simulink model "Test_1_2018a"  (Simulink 9.1)
settings: Solver=VariableStepAuto  StartTime=0.0  StopTime=32  RelTol=1e-3
values from neighbouring files (symbols this model uses):
  CdA = 0.08    [lqrparameters.m]
  d = 0.086    [lqrparameters.m]
  g = 9.81    [lqrparameters.m]
  Ix = 0.00025    [lqrparameters.m]
  Iy = 0.000432    [lqrparameters.m]
  Iz = 0.0003738    [lqrparameters.m]
  kfay = 0.01    [lqrparameters.m]
  kfaz = 0.01    [lqrparameters.m]
  kftx = 0.1    [lqrparameters.m]
  kfty = 0.1    [lqrparameters.m]
  kftz = 0.1    [lqrparameters.m]
  m = 0.18    [lqrparameters.m]
  rho = 1.225    [lqrparameters.m]
undefined symbols (not defined in the file or in its folder): DiscIntNeverNeededParam
libraries: peSlidingModeController x6, aerolibutil x1, sharedtransform x1, aerolibwind2 x1
settings Model: Creator=Ayush  LastModifiedBy=Rishabh Verma
settings DataIOCC: SaveFormat=Dataset
settings OptimizationCC: LifeSpan=auto
settings DebuggingCC: UnderspecifiedInitializationDetection=Simplified  MergeDetectMultiDrivingBlocksExec=error  LibraryContextMissingDiagnostic=warning  SFUnexpectedBacktrackingDiag=error  SFNoUnconditionalDefaultTransitionDiag=error  SFExecutionAtInitializationDiag=warning
settings HardwareCC: ProdBitPerPointer=64  ProdBitPerSizeT=64  ProdBitPerPtrDiffT=64  ProdLargestAtomicFloat=Float  ProdIntDivRoundTo=Zero  ProdEndianess=LittleEndian  ProdWordSize=64  ProdHWDeviceType=Intel->x86-64 (Windows64)
settings ModelReferenceCC: PropagateSignalLabelsOutOfModel=on
settings SFSimCC: SimUseLocalCustomCode=on
settings RTWCC: RTWUseLocalCustomCode=on
settings CodeAppCC: StateflowObjectComments=off
settings GRTTargetCC: TargetLangStandard=C99 (ISO)  CombineOutputUpdateFcns=on  GRTInterface=off
settings ConfigComp: CovMetricSettings=dwe  CovHtmlReporting=off  CovSaveCumulativeToWorkspaceVar=off  CovSaveSingleToWorkspaceVar=off  CovExternalEMLEnable=on

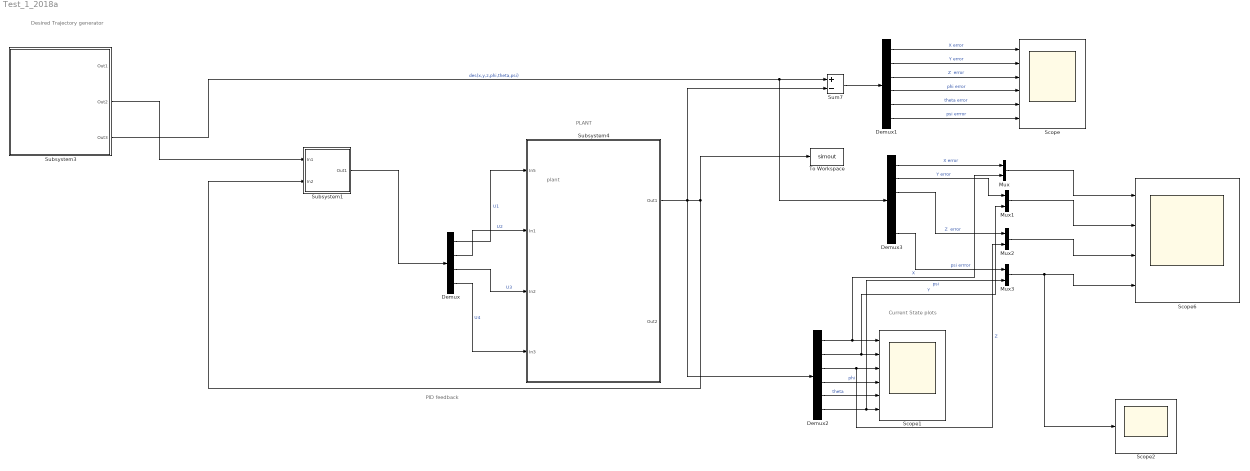
== system Test_1_2018a ==
  note: Desired Trajectory
      | generator
  note: PID feedback
  note: PLANT
  note: Current State
      | plots
  note: plant
  Demux : Demux
  Demux1 : Demux  Outputs=6
  Demux2 : Demux  Outputs=6
  Demux3 : Demux  Outputs=6
  Mux{,1..3} (4 alike) : Mux  Inputs=2
  Scope : Scope  NumInputPorts=6
  Scope1 : Scope  NumInputPorts=6
  Scope2 : Scope
  Scope6 : Scope  NumInputPorts=4
  Subsystem1 : Subsystem
  Subsystem3 : Subsystem
  Subsystem4 : Subsystem
  Sum7 : Sum  Inputs=+-
  To Workspace : ToWorkspace  VariableName=simout  SampleTime=0.01
  wires:
  Subsystem3/3(Out3) -> Demux3/1, Sum7/1  "des(x,y,z,phi,theta,psi)"
  Demux1/6 -> Scope/6  "psi errror"
  Demux1/5 -> Scope/5  "theta error"
  Demux1/2 -> Scope/2  "Y error"
  Sum7/1 -> Demux1/1
  Subsystem4/1(Out1) -> Sum7/2, Demux2/1, Subsystem1/2(In2), To Workspace/1
  Demux1/1 -> Scope/1  "X error"
  Demux2/4 -> Scope1/4  "phi"
  Demux2/1 -> Mux/2, Scope1/1  "X"
  Demux2/5 -> Scope1/5  "theta"
  Demux2/6 -> Mux3/2, Scope1/6  "psi"
  Demux2/3 -> Mux2/2, Scope1/3  "Z"
  Demux1/3 -> Scope/3  "Z  error"
  Demux2/2 -> Mux1/2, Scope1/2  "Y"
  Demux1/4 -> Scope/4  "phi error"
  Demux3/1 -> Mux/1  "X error"
  Demux3/2 -> Mux1/1  "Y error"
  Demux3/3 -> Mux2/1  "Z  error"
  Demux3/6 -> Mux3/1  "psi errror"
  Mux/1 -> Scope6/1
  Mux1/1 -> Scope6/2
  Mux2/1 -> Scope6/3
  Mux3/1 -> Scope2/1, Scope6/4
  Demux/1 -> Subsystem4/1(In5)  "U1"
  Demux/2 -> Subsystem4/2(In1)  "U2"
  Demux/3 -> Subsystem4/3(In2)  "U3"
  Demux/4 -> Subsystem4/4(In3)  "U4"
  Subsystem3/2(Out2) -> Subsystem1/1(In1)
  Subsystem1/1(Out1) -> Demux/1

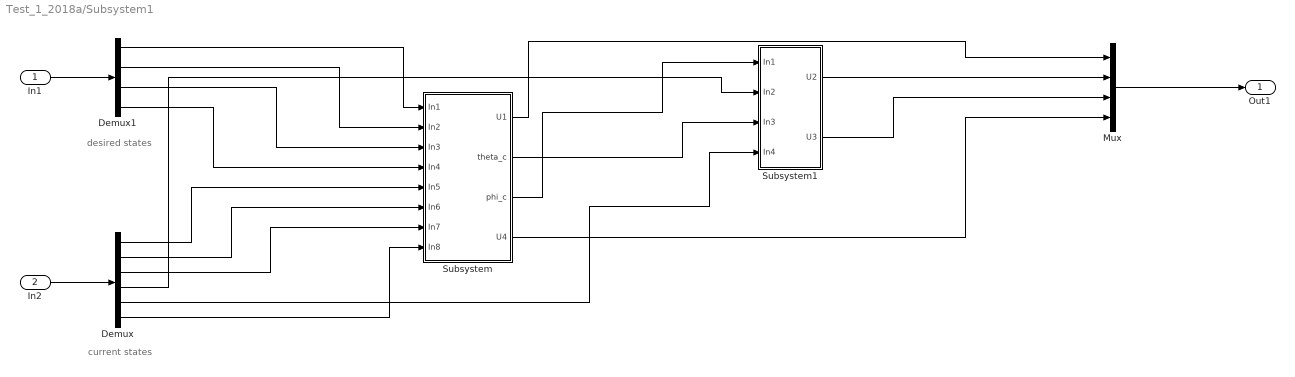
== system Test_1_2018a/Subsystem1 ==
  note: current states
  note: desired states
  In1 : Inport
  In2 : Inport  Port=2
  Demux : Demux  Outputs=6
  Demux1 : Demux
  Mux : Mux
  Subsystem : Subsystem
  Subsystem1 : Subsystem
  Out1 : Outport
  wires:
  Mux/1 -> Out1/1
  In2/1 -> Demux/1
  In1/1 -> Demux1/1
  Demux1/1 -> Subsystem/1(In1)
  Demux1/2 -> Subsystem/2(In2)
  Demux1/3 -> Subsystem/3(In3)
  Demux1/4 -> Subsystem/4(In4)
  Demux/1 -> Subsystem/5(In5)
  Demux/2 -> Subsystem/6(In6)
  Demux/3 -> Subsystem/7(In7)
  Demux/6 -> Subsystem/8(In8)
  Subsystem/2(theta_c) -> Subsystem1/3(In3)
  Demux/4 -> Subsystem1/2(In2)
  Demux/5 -> Subsystem1/4(In4)
  Subsystem/3(phi_c) -> Subsystem1/1(In1)
  Subsystem1/1(U2) -> Mux/2
  Subsystem/1(U1) -> Mux/1
  Subsystem/4(U4) -> Mux/4
  Subsystem1/2(U3) -> Mux/3

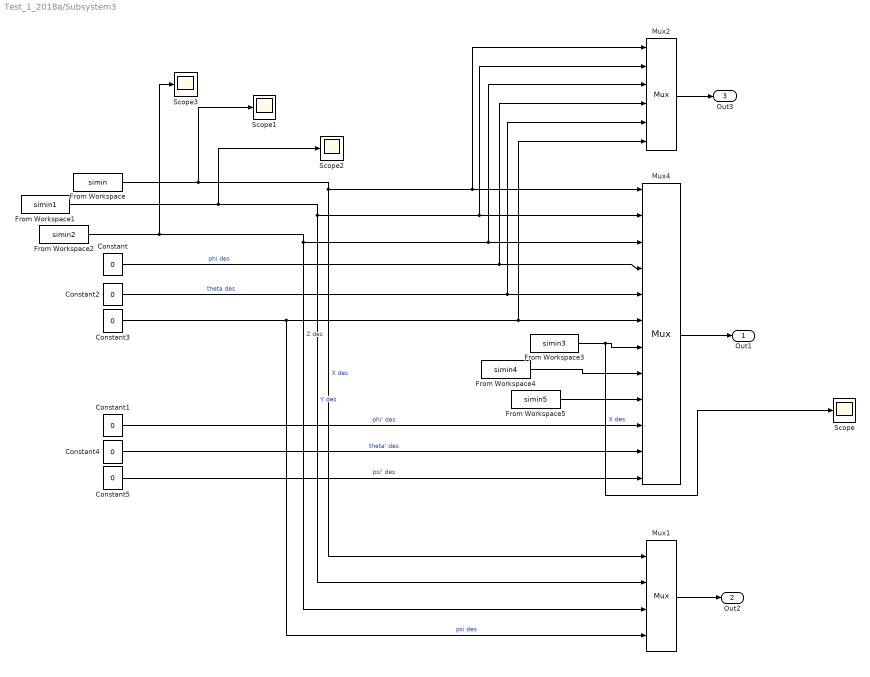
== system Test_1_2018a/Subsystem3 ==
  Constant{,1..5} (6 alike) : Constant  Value=0
  From Workspace : FromWorkspace  VariableName=simin  SampleTime=0
  From Workspace1 : FromWorkspace  VariableName=simin1  SampleTime=0
  From Workspace2 : FromWorkspace  VariableName=simin2  SampleTime=0
  From Workspace3 : FromWorkspace  VariableName=simin3  SampleTime=0
  From Workspace4 : FromWorkspace  VariableName=simin4  SampleTime=0
  From Workspace5 : FromWorkspace  VariableName=simin5  SampleTime=0
  Mux1 : Mux
      settings: DisplayOption=signals
  Mux2 : Mux  Inputs=6
      settings: DisplayOption=signals
  Mux4 : Mux  Inputs=12
      settings: DisplayOption=signals
  Scope{,1..3} (4 alike) : Scope
  Out1 : Outport
  Out2 : Outport  Port=2
  Out3 : Outport  Port=3
  wires:
  From Workspace/1 -> Scope1/1, Mux1/1, Mux2/1, Mux4/1  "X des"
  Constant1/1 -> Mux4/10  "phi' des"
  From Workspace1/1 -> Scope2/1, Mux1/2, Mux2/2, Mux4/2  "Y des"
  Constant2/1 -> Mux2/5, Mux4/5  "theta des"
  Constant/1 -> Mux2/4, Mux4/4  "phi des"
  Constant5/1 -> Mux4/12  "psi' des"
  From Workspace2/1 -> Scope3/1, Mux1/3, Mux2/3, Mux4/3  "Z des"
  Constant3/1 -> Mux1/4, Mux2/6, Mux4/6  "psi des"
  Constant4/1 -> Mux4/11  "theta' des"
  Mux1/1 -> Out2/1
  Mux4/1 -> Out1/1
  Mux2/1 -> Out3/1
  From Workspace4/1 -> Mux4/8
  From Workspace5/1 -> Mux4/9
  From Workspace3/1 -> Scope/1, Mux4/7  "X des"

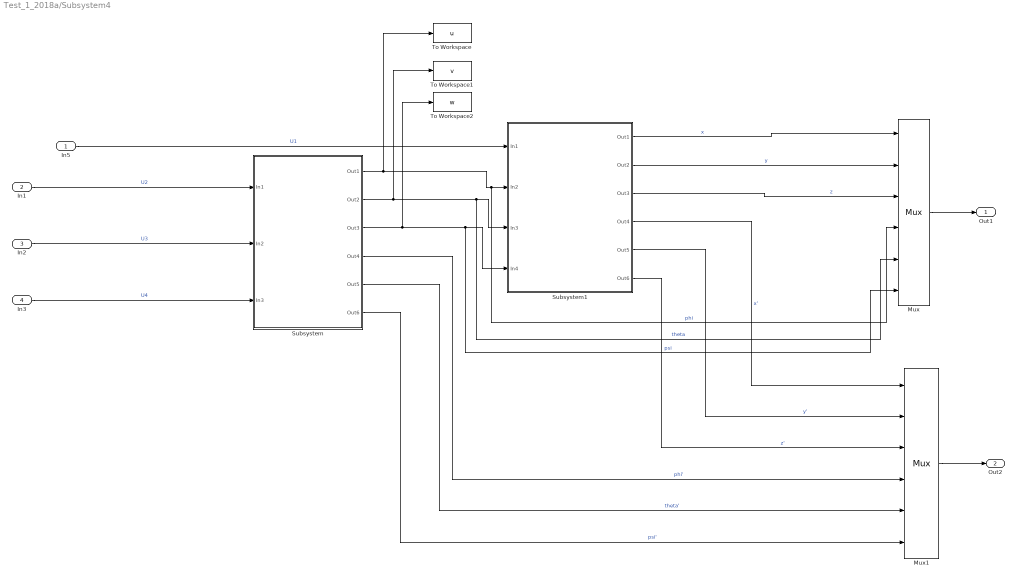
== system Test_1_2018a/Subsystem4 ==
  In5 : Inport
  In1 : Inport  Port=2
  In2 : Inport  Port=3
  In3 : Inport  Port=4
  Mux : Mux  Inputs=6
      settings: DisplayOption=signals
  Mux1 : Mux  Inputs=6
      settings: DisplayOption=signals
  Subsystem : Subsystem
  Subsystem1 : Subsystem
  To Workspace : ToWorkspace  VariableName=u  SaveFormat=Timeseries  SampleTime=-1
  To Workspace1 : ToWorkspace  VariableName=v  SaveFormat=Timeseries  SampleTime=-1
  To Workspace2 : ToWorkspace  VariableName=w  SaveFormat=Timeseries  SampleTime=-1
  Out1 : Outport
  Out2 : Outport  Port=2
  wires:
  Subsystem1/2(Out2) -> Mux/2  "y"
  Subsystem/1(Out1) -> To Workspace/1, Subsystem1/2(In2), Mux/4  "phi"
  Subsystem1/1(Out1) -> Mux/1  "x"
  In1/1 -> Subsystem/1(In1)  "U2"
  Subsystem/3(Out3) -> To Workspace2/1, Mux/6, Subsystem1/4(In4)  "psi"
  In3/1 -> Subsystem/3(In3)  "U4"
  Subsystem1/3(Out3) -> Mux/3  "z"
  Subsystem1/6(Out6) -> Mux1/3  "z'"
  In2/1 -> Subsystem/2(In2)  "U3"
  In5/1 -> Subsystem1/1(In1)  "U1"
  Subsystem1/4(Out4) -> Mux1/1  "x'"
  Subsystem1/5(Out5) -> Mux1/2  "y'"
  Subsystem/2(Out2) -> To Workspace1/1, Mux/5, Subsystem1/3(In3)  "theta"
  Subsystem/4(Out4) -> Mux1/4  "phi'"
  Subsystem/5(Out5) -> Mux1/5  "theta'"
  Subsystem/6(Out6) -> Mux1/6  "psi'"
  Mux/1 -> Out1/1
  Mux1/1 -> Out2/1

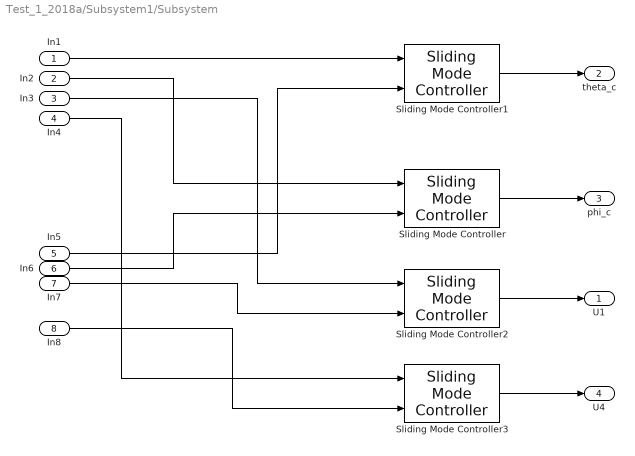
== system Test_1_2018a/Subsystem1/Subsystem ==
  In1 : Inport
  In2 : Inport  Port=2
  In3 : Inport  Port=3
  In4 : Inport  Port=4
  In5 : Inport  Port=5
  In6 : Inport  Port=6
  In7 : Inport  Port=7
  In8 : Inport  Port=8
  Sliding Mode Controller{,1..3} (4 alike) : peSlidingModeController/Sliding Mode Controller  h=0.2  up=10  lo=-10  Ts=-1
  U1 : Outport
  theta_c : Outport  Port=2
  phi_c : Outport  Port=3
  U4 : Outport  Port=4
  wires:
  In6/1 -> Sliding Mode Controller/2
  In1/1 -> Sliding Mode Controller1/1
  In7/1 -> Sliding Mode Controller2/2
  In5/1 -> Sliding Mode Controller1/2
  In4/1 -> Sliding Mode Controller3/1
  In2/1 -> Sliding Mode Controller/1
  In3/1 -> Sliding Mode Controller2/1
  In8/1 -> Sliding Mode Controller3/2
  Sliding Mode Controller2/1 -> U1/1
  Sliding Mode Controller3/1 -> U4/1
  Sliding Mode Controller1/1 -> theta_c/1
  Sliding Mode Controller/1 -> phi_c/1

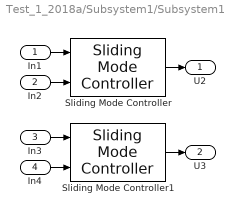
== system Test_1_2018a/Subsystem1/Subsystem1 ==
  In1 : Inport
  In2 : Inport  Port=2
  In3 : Inport  Port=3
  In4 : Inport  Port=4
  Sliding Mode Controller : peSlidingModeController/Sliding Mode Controller  h=0.2  up=10  lo=-10  Ts=-1
  Sliding Mode Controller1 : peSlidingModeController/Sliding Mode Controller  h=0.2  up=10  lo=-10  Ts=-1
  U2 : Outport
  U3 : Outport  Port=2
  wires:
  Sliding Mode Controller1/1 -> U3/1
  In2/1 -> Sliding Mode Controller/2
  In3/1 -> Sliding Mode Controller1/1
  In4/1 -> Sliding Mode Controller1/2
  Sliding Mode Controller/1 -> U2/1
  In1/1 -> Sliding Mode Controller/1

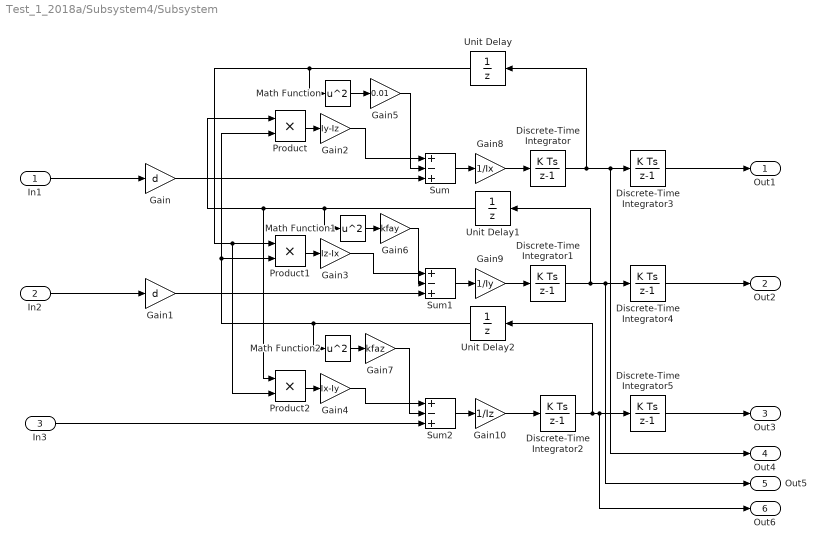
== system Test_1_2018a/Subsystem4/Subsystem ==
  In1 : Inport
  In2 : Inport  Port=2
  In3 : Inport  Port=3
  Discrete-Time Integrator{,1..5} (6 alike) : DiscreteIntegrator  SampleTime=-1  ICPrevOutput=DiscIntNeverNeededParam  ICPrevScaledInput=DiscIntNeverNeededParam
  Gain : Gain  Gain=d
  Gain1 : Gain  Gain=d
  Gain10 : Gain  Gain=1/Iz
  Gain2 : Gain  Gain=Iy-Iz
  Gain3 : Gain  Gain=Iz-Ix
  Gain4 : Gain  Gain=Ix-Iy
  Gain5 : Gain  Gain=0.01
  Gain6 : Gain  Gain=kfay
  Gain7 : Gain  Gain=kfaz
  Gain8 : Gain  Gain=1/Ix
  Gain9 : Gain  Gain=1/Iy
  Math Function : Math  Operator=square  SaturateOnIntegerOverflow=on
  Math Function1 : Math  Operator=square  SaturateOnIntegerOverflow=on
  Math Function2 : Math  Operator=square  SaturateOnIntegerOverflow=on
  Product : Product
  Product1 : Product
  Product2 : Product
  Sum : Sum  Inputs=+-+
  Sum1 : Sum  Inputs=+-+
  Sum2 : Sum  Inputs=+-+
  Unit Delay : UnitDelay  SampleTime=0.001
  Unit Delay1 : UnitDelay  SampleTime=0.001
  Unit Delay2 : UnitDelay  SampleTime=0.001
  Out1 : Outport
  Out2 : Outport  Port=2
  Out3 : Outport  Port=3
  Out4 : Outport  Port=4
  Out5 : Outport  Port=5
  Out6 : Outport  Port=6
  wires:
  Unit Delay/1 -> Math Function/1, Product2/2, Product1/1
  Discrete-Time Integrator1/1 -> Out5/1, Discrete-Time Integrator4/1, Unit Delay1/1
  Unit Delay1/1 -> Math Function1/1, Product2/1, Product/1
  Discrete-Time Integrator2/1 -> Out6/1, Discrete-Time Integrator5/1, Unit Delay2/1
  Unit Delay2/1 -> Math Function2/1, Product1/2, Product/2
  Product1/1 -> Gain3/1
  Discrete-Time Integrator/1 -> Out4/1, Discrete-Time Integrator3/1, Unit Delay/1
  Gain10/1 -> Discrete-Time Integrator2/1
  Discrete-Time Integrator3/1 -> Out1/1
  Gain4/1 -> Sum2/1
  Gain/1 -> Sum/3
  Discrete-Time Integrator4/1 -> Out2/1
  Math Function/1 -> Gain5/1
  Gain5/1 -> Sum/2
  Product/1 -> Gain2/1
  Math Function1/1 -> Gain6/1
  Gain6/1 -> Sum1/2
  Gain7/1 -> Sum2/2
  Gain2/1 -> Sum/1
  Math Function2/1 -> Gain7/1
  Sum2/1 -> Gain10/1
  Gain9/1 -> Discrete-Time Integrator1/1
  Gain8/1 -> Discrete-Time Integrator/1
  Sum/1 -> Gain8/1
  Gain3/1 -> Sum1/1
  Product2/1 -> Gain4/1
  Gain1/1 -> Sum1/3
  Sum1/1 -> Gain9/1
  Discrete-Time Integrator5/1 -> Out3/1
  In1/1 -> Gain/1
  In2/1 -> Gain1/1
  In3/1 -> Sum2/3

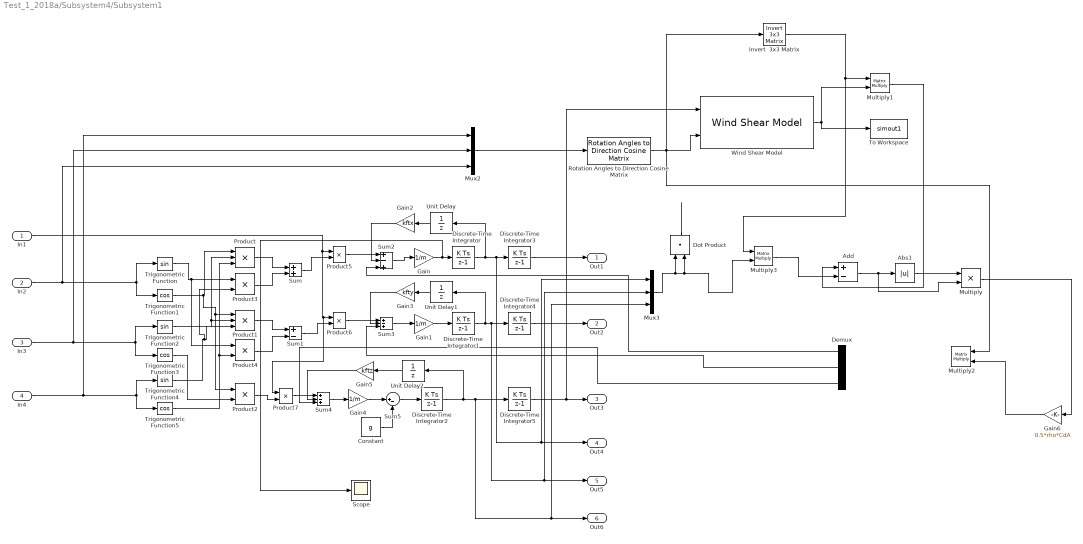
== system Test_1_2018a/Subsystem4/Subsystem1 ==
  In1 : Inport
  In2 : Inport  Port=2
  In3 : Inport  Port=3
  In4 : Inport  Port=4
  Abs1 : Abs
  Add : Sum  Inputs=+-
  Constant : Constant  Value=g
  Demux : Demux  Outputs=3
  Discrete-Time Integrator{,1..5} (6 alike) : DiscreteIntegrator  SampleTime=0.001  ICPrevOutput=DiscIntNeverNeededParam  ICPrevScaledInput=DiscIntNeverNeededParam
  Dot Product : DotProduct  InputSameDT=on  OutDataTypeStr=Inherit: Inherit via internal rule
  Gain : Gain  Gain=1/m
  Gain1 : Gain  Gain=1/m
  Gain2 : Gain  Gain=kftx
  Gain3 : Gain  Gain=kfty
  Gain4 : Gain  Gain=1/m
  Gain5 : Gain  Gain=kftz
  Gain6 : Gain  Gain=0.5*rho*CdA
  Invert  3x3 Matrix : aerolibutil/Invert  3x3 Matrix
  Multiply : Product
  Multiply1 : Product  Multiplication=Matrix(*)
  Multiply2 : Product  Multiplication=Matrix(*)
  Multiply3 : Product  Multiplication=Matrix(*)
  Mux2 : Mux  Inputs=3
  Mux3 : Mux  Inputs=3
  Product : Product  Inputs=3
  Product1 : Product  Inputs=3
  Product{2..7} (6 alike) : Product
  Rotation Angles to Direction Cosine Matrix : sharedtransform/Rotation Angles to Direction Cosine Matrix  rotationOrder=XYZ  aMode=aMode
      settings: SourceProductBaseCode=AE
  Scope : Scope
  Sum : Sum
  Sum1 : Sum  Inputs=+-
  Sum2 : Sum  Inputs=+-+
  Sum3 : Sum  Inputs=+-+
  Sum4 : Sum  Inputs=+-+
  Sum5 : Sum  Inputs=|+-
  To Workspace : ToWorkspace  VariableName=simout1  SampleTime=0.01
  Trigonometric Function : Trigonometry
  Trigonometric Function1 : Trigonometry  Operator=cos
  Trigonometric Function2 : Trigonometry
  Trigonometric Function3 : Trigonometry  Operator=cos
  Trigonometric Function4 : Trigonometry
  Trigonometric Function5 : Trigonometry  Operator=cos
  Unit Delay : UnitDelay  SampleTime=0.001
  Unit Delay1 : UnitDelay  SampleTime=0.001
  Unit Delay2 : UnitDelay  SampleTime=0.001
  Wind Shear Model : aerolibwind2/Wind Shear Model  units=Metric (MKS)  phase=Category C - Terminal Flight Phase  W_20=8.5  Wdeg=0
      settings: SourceProductName=Aerospace Blockset
  Out1 : Outport
  Out2 : Outport  Port=2
  Out3 : Outport  Port=3
  Out4 : Outport  Port=4
  Out5 : Outport  Port=5
  Out6 : Outport  Port=6
  wires:
  Sum2/1 -> Gain/1
  Trigonometric Function2/1 -> Product/2, Product1/2
  Unit Delay/1 -> Gain2/1
  Discrete-Time Integrator2/1 -> Mux3/3, Out6/1, Discrete-Time Integrator5/1, Unit Delay2/1
  Gain5/1 -> Sum4/2
  Trigonometric Function4/1 -> Product3/2, Product1/3
  Trigonometric Function1/1 -> Product2/1, Product1/1, Product/1
  Product3/1 -> Sum/2
  Gain/1 -> Scope/1, Discrete-Time Integrator/1
  Product/1 -> Sum/1
  Sum5/1 -> Discrete-Time Integrator2/1
  Sum1/1 -> Product6/2
  Sum/1 -> Product5/2
  Product6/1 -> Sum3/1
  Discrete-Time Integrator1/1 -> Mux3/2, Out5/1, Discrete-Time Integrator4/1, Unit Delay1/1
  In1/1 -> Product7/1, Product6/1, Product5/1
  Constant/1 -> Sum5/2
  Discrete-Time Integrator/1 -> Mux3/1, Out4/1, Discrete-Time Integrator3/1, Unit Delay/1
  In3/1 -> Mux2/2, Trigonometric Function2/1, Trigonometric Function3/1
  Sum4/1 -> Gain4/1
  Gain4/1 -> Sum5/1
  Unit Delay1/1 -> Gain3/1
  Trigonometric Function5/1 -> Product4/2, Product/3
  Trigonometric Function/1 -> Product4/1, Product3/1
  In2/1 -> Mux2/3, Trigonometric Function/1, Trigonometric Function1/1
  Discrete-Time Integrator3/1 -> Out1/1
  Unit Delay2/1 -> Gain5/1
  Gain1/1 -> Discrete-Time Integrator1/1
  Sum3/1 -> Gain1/1
  Product5/1 -> Sum2/1
  Gain3/1 -> Sum3/2
  Gain2/1 -> Sum2/2
  Trigonometric Function3/1 -> Product2/2
  Product4/1 -> Sum1/2
  Product1/1 -> Sum1/1
  Discrete-Time Integrator4/1 -> Out2/1
  Discrete-Time Integrator5/1 -> Wind Shear Model/1, Out3/1
  Product2/1 -> Product7/2
  Product7/1 -> Sum4/1
  Rotation Angles to Direction Cosine Matrix/1 -> Wind Shear Model/2, Multiply2/1, Invert  3x3 Matrix/1
  In4/1 -> Mux2/1, Trigonometric Function4/1, Trigonometric Function5/1
  Dot Product/1 -> ?
  Multiply1/1 -> Add/1
  Mux3/1 -> Dot Product/1, Dot Product/2, Multiply3/2
  Abs1/1 -> Multiply/1
  Add/1 -> Abs1/1, Multiply/2
  Multiply/1 -> Gain6/1
  Gain6/1 -> Multiply2/2
  Invert  3x3 Matrix/1 -> Multiply3/1, Multiply1/1
  Multiply3/1 -> Add/2
  Mux2/1 -> Rotation Angles to Direction Cosine Matrix/1
  Wind Shear Model/1 -> To Workspace/1, Multiply1/2
  Demux/1 -> Sum2/3
  Demux/2 -> Sum3/3
  Demux/3 -> Sum4/3
